simulink model "phys3011"  (R2024a)
settings: Solver=VariableStepAuto  StartTime=0.0  StopTime=150.0  RelTol=1e-3
settings Model: Creator=pupkinzalupkin  LastModifiedBy=pupkinzalupkin

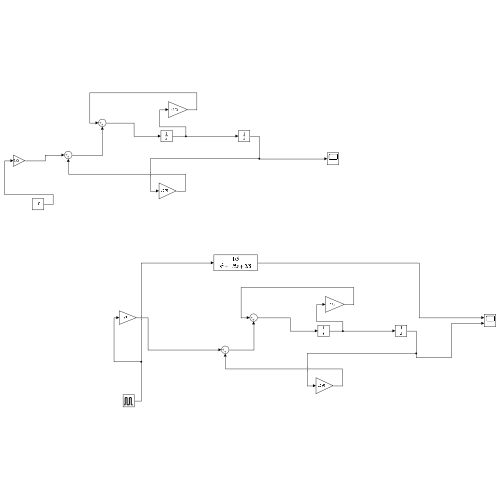
[thumbnail: Simulink's stored preview of the top-level diagram]
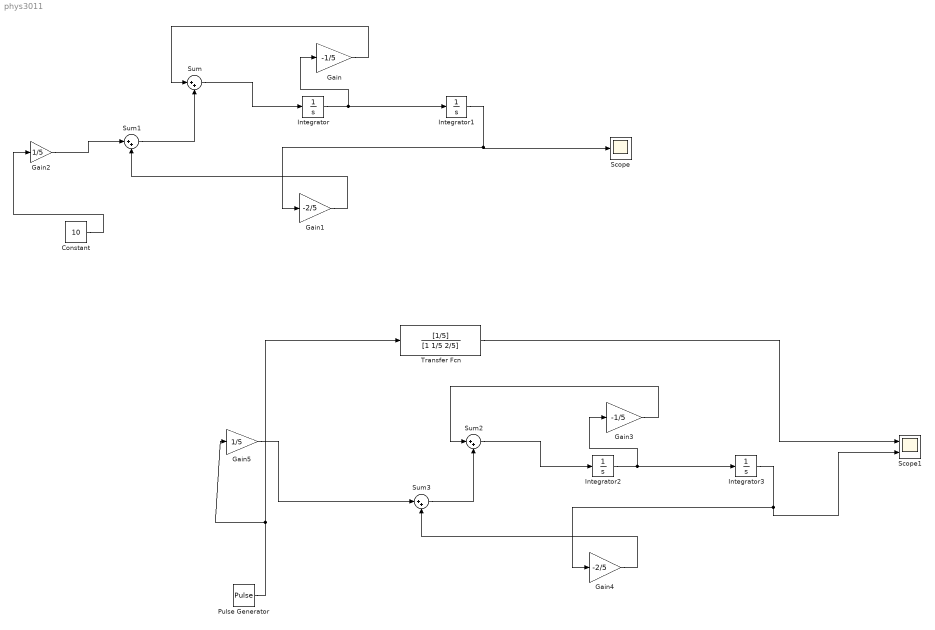
== system phys3011 ==
  Constant : Constant  Value=10
  Gain : Gain  Gain=-1/5
  Gain1 : Gain  Gain=-2/5
  Gain2 : Gain  Gain=1/5
  Gain3 : Gain  Gain=-1/5
  Gain4 : Gain  Gain=-2/5
  Gain5 : Gain  Gain=1/5
  Integrator : Integrator
  Integrator1 : Integrator  InitialCondition=1
  Integrator2 : Integrator
  Integrator3 : Integrator
  Pulse Generator : DiscretePulseGenerator  PulseType=Time based  Period=100  PulseWidth=5  PhaseDelay=20
  Scope : Scope
  Scope1 : Scope  NumInputPorts=2
  Sum{,1..3} (4 alike) : Sum  Inputs=|++
  Transfer Fcn : TransferFcn  Numerator=[1/5]  Denominator=[1 1/5 2/5]
  wires:
  Integrator/1 -> Integrator1/1, Gain/1
  Integrator1/1 -> Scope/1, Gain1/1
  Gain/1 -> Sum/1
  Sum/1 -> Integrator/1
  Gain1/1 -> Sum1/2
  Sum1/1 -> Sum/2
  Constant/1 -> Gain2/1
  Gain2/1 -> Sum1/1
  Integrator3/1 -> Scope1/2, Gain4/1
  Integrator2/1 -> Integrator3/1, Gain3/1
  Sum3/1 -> Sum2/2
  Gain3/1 -> Sum2/1
  Gain5/1 -> Sum3/1
  Gain4/1 -> Sum3/2
  Sum2/1 -> Integrator2/1
  Transfer Fcn/1 -> Scope1/1
  Pulse Generator/1 -> Gain5/1, Transfer Fcn/1
